simulink model "DDMRmodel"  (R2018a)
settings: Solver=VariableStepAuto  StartTime=0.0  StopTime=10.0  RelTol=1e-3
values from neighbouring files (symbols this model uses):
  d = 0.0445    [DDMRsimulinkParameters.m]    (also in Params.m = 1; dataSimulink.mat; p3dx_constants.m = 0.381)
  J = M*1.2e-1    (= 1.08)    [DDMRsimulinkParameters.m]    (also in Params.m = 1; dataSimulink.mat = 0.192; p3dx_constants.m = 0.2641395)
  L = 0.1655    [DDMRsimulinkParameters.m]    (also in Params.m = 1; dataSimulink.mat; p3dx_constants.m = 0.381)
  M = 9    [DDMRsimulinkParameters.m]    (also in Params.m = 1; dataSimulink.mat = 1.6; p3dx_constants.m)
  R = 195e-3/2    (= 0.0975)    [DDMRsimulinkParameters.m]    (also in Params.m = 1; dataSimulink.mat = 0.097541; p3dx_constants.m)
settings Model: Creator=Egydio Tadeu  LastModifiedBy=Egydio Tadeu

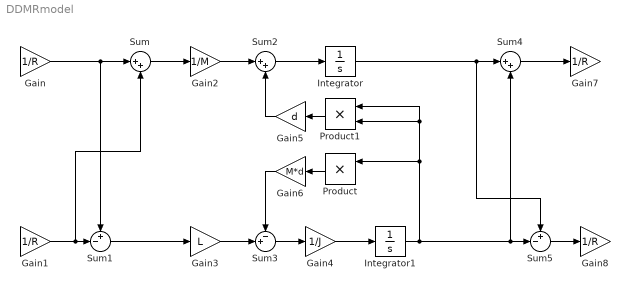
== system DDMRmodel ==
  Gain{,1,7..8} (4 alike) : Gain  Gain=1/R
  Gain2 : Gain  Gain=1/M
  Gain3 : Gain  Gain=L
  Gain4 : Gain  Gain=1/J
  Gain5 : Gain  Gain=d
  Gain6 : Gain  Gain=M*d
  Integrator : Integrator
  Integrator1 : Integrator
  Product : Product
  Product1 : Product
  Sum : Sum  Inputs=|++
  Sum1 : Sum  Inputs=+-|
  Sum2 : Sum  Inputs=|++
  Sum3 : Sum  Inputs=-+|
  Sum4 : Sum  Inputs=|++
  Sum5 : Sum  Inputs=+-|
  wires:
  Gain/1 -> Sum1/1, Sum/1
  Gain1/1 -> Sum/2, Sum1/2
  Sum/1 -> Gain2/1
  Sum1/1 -> Gain3/1
  Gain2/1 -> Sum2/1
  Gain3/1 -> Sum3/2
  Sum3/1 -> Gain4/1
  Sum2/1 -> Integrator/1
  Gain4/1 -> Integrator1/1
  Product1/1 -> Gain5/1
  Gain5/1 -> Sum2/2
  Product/1 -> Gain6/1
  Gain6/1 -> Sum3/1
  Integrator1/1 -> Sum4/2, Sum5/2, Product/1, Product1/1, Product1/2
  Integrator/1 -> Sum4/1, Sum5/1
  Sum4/1 -> Gain7/1
  Sum5/1 -> Gain8/1
